simulink model "simu_21a"  (R2021a)
settings: Solver=VariableStepAuto  StartTime=0.0  StopTime=10.0  RelTol=1e-3
settings Model: Creator=psp_dada  LastModifiedBy=psp_dada
settings DebuggingCC: UnconnectedInputMsg=none  UnconnectedOutputMsg=none  UnconnectedLineMsg=none
settings ModelReferenceCC: EnableRefExpFcnMdlSchedulingChecks=off
settings RTWCC: Description=Generic Real-Time Target  GPUComputeCapability=5.0  DLArmComputeVersion=20.02.1
settings ConfigComp: CovBoundaryAbsTol=1.0e-5

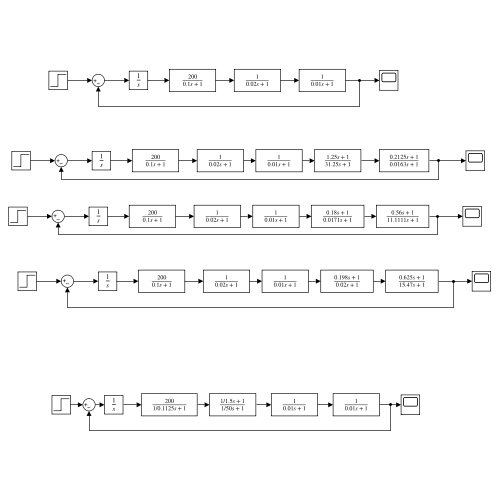
[thumbnail: Simulink's stored preview of the top-level diagram]
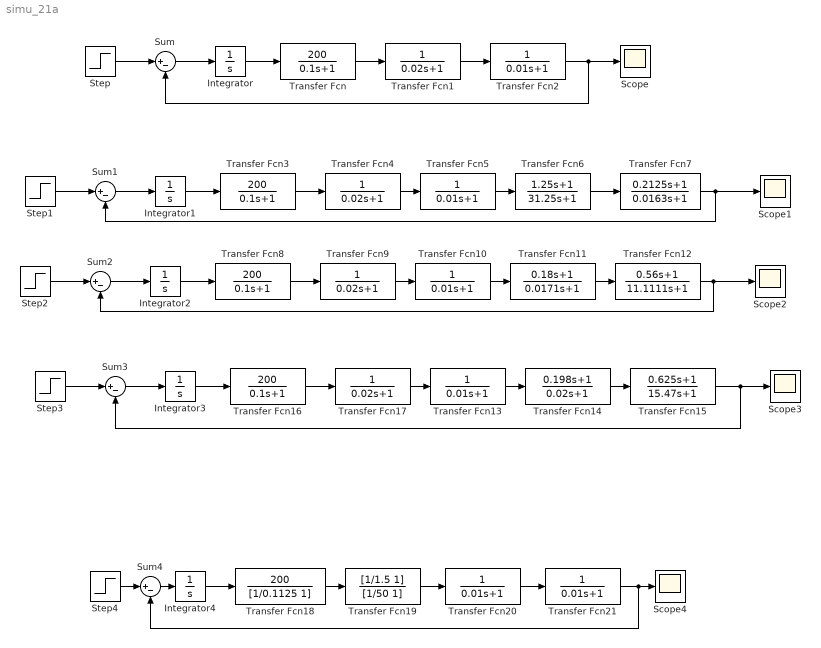
== system simu_21a ==
  Integrator{,1..4} (5 alike) : Integrator
  Scope{,1..4} (5 alike) : Scope
  Step{,1..4} (5 alike) : Step  SampleTime=0
  Sum{,1..4} (5 alike) : Sum  Inputs=|+-
  Transfer Fcn{,3,8,16} (4 alike) : TransferFcn  Numerator=[200]  Denominator=[0.1 1]
  Transfer Fcn{1,4,9,17} (4 alike) : TransferFcn  Denominator=[0.02 1]
  Transfer Fcn{2,5,10,13,20..21} (6 alike) : TransferFcn  Denominator=[0.01 1]
  Transfer Fcn11 : TransferFcn  Numerator=[0.18 1]  Denominator=[0.0171 1]
  Transfer Fcn12 : TransferFcn  Numerator=[0.56 1]  Denominator=[11.1111 1]
  Transfer Fcn14 : TransferFcn  Numerator=[0.198 1]  Denominator=[0.02 1]
  Transfer Fcn15 : TransferFcn  Numerator=[0.625 1]  Denominator=[15.47 1]
  Transfer Fcn18 : TransferFcn  Numerator=[200]  Denominator=[1/0.1125 1]
  Transfer Fcn19 : TransferFcn  Numerator=[1/1.5 1]  Denominator=[1/50 1]
  Transfer Fcn6 : TransferFcn  Numerator=[1.25 1]  Denominator=[31.25 1]
  Transfer Fcn7 : TransferFcn  Numerator=[0.2125 1]  Denominator=[0.0163 1]
  wires:
  Step/1 -> Sum/1
  Integrator/1 -> Transfer Fcn/1
  Transfer Fcn/1 -> Transfer Fcn1/1
  Transfer Fcn1/1 -> Transfer Fcn2/1
  Sum/1 -> Integrator/1
  Transfer Fcn2/1 -> Sum/2, Scope/1
  Transfer Fcn4/1 -> Transfer Fcn5/1
  Step1/1 -> Sum1/1
  Transfer Fcn3/1 -> Transfer Fcn4/1
  Transfer Fcn7/1 -> Sum1/2, Scope1/1
  Sum1/1 -> Integrator1/1
  Integrator1/1 -> Transfer Fcn3/1
  Transfer Fcn5/1 -> Transfer Fcn6/1
  Transfer Fcn6/1 -> Transfer Fcn7/1
  Transfer Fcn11/1 -> Transfer Fcn12/1
  Transfer Fcn12/1 -> Sum2/2, Scope2/1
  Transfer Fcn10/1 -> Transfer Fcn11/1
  Transfer Fcn9/1 -> Transfer Fcn10/1
  Integrator2/1 -> Transfer Fcn8/1
  Step2/1 -> Sum2/1
  Transfer Fcn8/1 -> Transfer Fcn9/1
  Sum2/1 -> Integrator2/1
  Step3/1 -> Sum3/1
  Transfer Fcn13/1 -> Transfer Fcn14/1
  Transfer Fcn17/1 -> Transfer Fcn13/1
  Transfer Fcn15/1 -> Sum3/2, Scope3/1
  Transfer Fcn14/1 -> Transfer Fcn15/1
  Sum3/1 -> Integrator3/1
  Transfer Fcn16/1 -> Transfer Fcn17/1
  Integrator3/1 -> Transfer Fcn16/1
  Transfer Fcn19/1 -> Transfer Fcn20/1
  Step4/1 -> Sum4/1
  Transfer Fcn18/1 -> Transfer Fcn19/1
  Transfer Fcn21/1 -> Sum4/2, Scope4/1
  Sum4/1 -> Integrator4/1
  Integrator4/1 -> Transfer Fcn18/1
  Transfer Fcn20/1 -> Transfer Fcn21/1
